simulink model "DisableController"  (Simulink 8.6)
settings: Solver=VariableStepAuto  StartTime=0.0  StopTime=inf  RelTol=1e-3
libraries: simulink_extras x1
settings Model: Creator=Oscar  LastModifiedBy=Oscar
settings DataIOCC: SaveFormat=Dataset  SignalLoggingSaveFormat=Dataset
settings OptimizationCC: ExpressionDepthLimit=128
settings DebuggingCC: UnderspecifiedInitializationDetection=Simplified  MergeDetectMultiDrivingBlocksExec=error  SolverPrmCheckMsg=none  FcnCallInpInsideContextMsg=EnableAllAsError  StateNameClashWarn=none
settings HardwareCC: ProdBitPerPointer=64  ProdLargestAtomicFloat=Float  ProdIntDivRoundTo=Zero  ProdEndianess=LittleEndian  ProdWordSize=64  ProdHWDeviceType=Intel->x86-64 (Windows64)
settings GRTTargetCC: GeneratePreprocessorConditionals=Use local settings  CombineOutputUpdateFcns=on  GRTInterface=off
settings ConfigComp: CovModelRefEnable=off

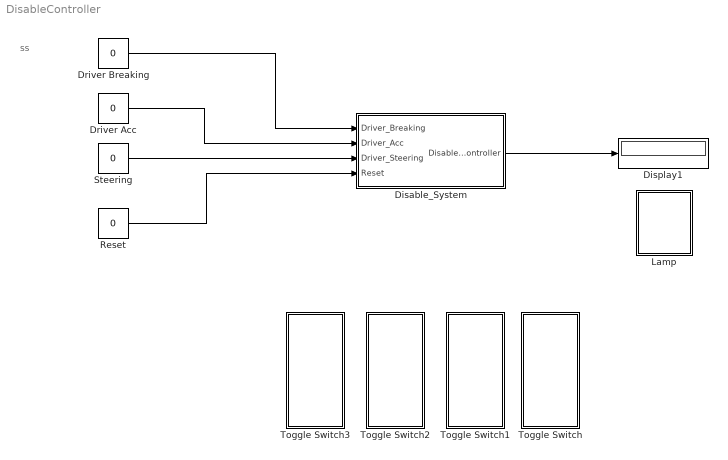
== system DisableController ==
  note: ss
  Disable_System : Subsystem
  Display1 : Display
  Driver Acc : Constant  Value=0
  Driver Breaking : Constant  Value=0
  Lamp : Subsystem  DialogController=hmiCreateDDGDialog  DialogControllerArgs=DataTag0  IsWebBlock=on  mask(MWDashboardBlock){webBlockId=f0d4b18d-8bb7-414d-912f-2697fe4de823, webBlockType=lamp, ShowInLibBrowser=on, ShowInitialText=on, HMISrcModelName=DisableController}
      mask prompts: webBlockType "WebBlock Type"; HMISrcModelName "Source Model"
      mask Help: helpview([docroot '/mapfiles/simulink.map'], 'hmi_lamp')
      mask Display:
      | if strcmp(get_param(bdroot(gcb),'BlockDiagramType'), 'library')
      |     image([(matlabroot) '/toolbox/simulink/hmi/icons/Lamp.png']);
      | end
  Reset : Constant  Value=0
  Steering : Constant  Value=0
  Toggle Switch : Subsystem  DialogController=hmiCreateDDGDialog  DialogControllerArgs=DataTag1  IsWebBlock=on  mask(MWDashboardBlock){webBlockId=8696f94f-6ba7-4cf2-b2c4-95ca151c8475, webBlockType=toggleswitch, ShowInLibBrowser=on, ShowInitialText=on, HMISrcModelName=DisableController}
      mask prompts: webBlockId "WebBlock Id"; webBlockType "WebBlock Type"; HMISrcModelName "Source Model"
      mask Help: helpview([docroot '/mapfiles/simulink.map'], 'hmi_toggle_switch')
      mask Display:
      | if strcmp(get_param(bdroot(gcb),'BlockDiagramType'), 'library')
      |     image([(matlabroot) '/toolbox/simulink/hmi/icons/ToggleSwitch.png']);
      | end
  Toggle Switch1 : Subsystem  DialogController=hmiCreateDDGDialog  DialogControllerArgs=DataTag2  IsWebBlock=on  mask(MWDashboardBlock){webBlockId=361f9ab1-9628-4675-8173-fcd33670bfa1, webBlockType=toggleswitch, ShowInLibBrowser=on, ShowInitialText=on, HMISrcModelName=DisableController}
      mask prompts: webBlockId "WebBlock Id"; webBlockType "WebBlock Type"; HMISrcModelName "Source Model"
      mask Help: helpview([docroot '/mapfiles/simulink.map'], 'hmi_toggle_switch')
      mask Display:
      | if strcmp(get_param(bdroot(gcb),'BlockDiagramType'), 'library')
      |     image([(matlabroot) '/toolbox/simulink/hmi/icons/ToggleSwitch.png']);
      | end
  Toggle Switch2 : Subsystem  DialogController=hmiCreateDDGDialog  DialogControllerArgs=DataTag3  IsWebBlock=on  mask(MWDashboardBlock){webBlockId=eedc1ba2-2433-4e35-ba26-c33148832a6b, webBlockType=toggleswitch, ShowInLibBrowser=on, ShowInitialText=on, HMISrcModelName=DisableController}
      mask prompts: webBlockId "WebBlock Id"; webBlockType "WebBlock Type"; HMISrcModelName "Source Model"
      mask Help: helpview([docroot '/mapfiles/simulink.map'], 'hmi_toggle_switch')
      mask Display:
      | if strcmp(get_param(bdroot(gcb),'BlockDiagramType'), 'library')
      |     image([(matlabroot) '/toolbox/simulink/hmi/icons/ToggleSwitch.png']);
      | end
  Toggle Switch3 : Subsystem  DialogController=hmiCreateDDGDialog  DialogControllerArgs=DataTag4  IsWebBlock=on  mask(MWDashboardBlock){webBlockId=0cae81f2-8a2d-4286-bc79-44c17df7e163, webBlockType=toggleswitch, ShowInLibBrowser=on, ShowInitialText=on, HMISrcModelName=DisableController}
      mask prompts: webBlockId "WebBlock Id"; webBlockType "WebBlock Type"; HMISrcModelName "Source Model"
      mask Help: helpview([docroot '/mapfiles/simulink.map'], 'hmi_toggle_switch')
      mask Display:
      | if strcmp(get_param(bdroot(gcb),'BlockDiagramType'), 'library')
      |     image([(matlabroot) '/toolbox/simulink/hmi/icons/ToggleSwitch.png']);
      | end
  wires:
  Driver Breaking/1 -> Disable_System/1(Driver_Breaking)
  Driver Acc/1 -> Disable_System/2(Driver_Acc)
  Reset/1 -> Disable_System/4(Reset)
  Disable_System/1(Disable_Controller) -> Display1/1
  Steering/1 -> Disable_System/3(Driver_Steering)

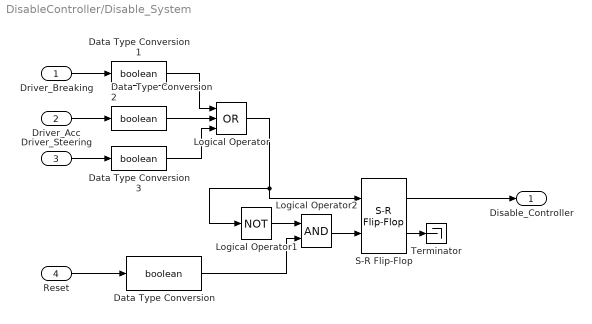
== system DisableController/Disable_System ==
  Driver_Breaking : Inport
  Driver_Acc : Inport  Port=2
  Driver_Steering : Inport  Port=3
  Reset : Inport  Port=4
  Data Type Conversion{,1..3} (4 alike) : DataTypeConversion  OutDataTypeStr=boolean
  Logical Operator : Logic  Operator=OR  Inputs=3  AllPortsSameDT=off  OutDataTypeStr=boolean
  Logical Operator1 : Logic  Operator=NOT  AllPortsSameDT=off  OutDataTypeStr=boolean
  Logical Operator2 : Logic  AllPortsSameDT=off  OutDataTypeStr=boolean
  S-R Flip-Flop : simulink_extras/Flip Flops/S-R Flip-Flop  initial_condition=0
  Terminator : Terminator
  Disable_Controller : Outport
  wires:
  Logical Operator1/1 -> Logical Operator2/1
  Driver_Acc/1 -> Data Type Conversion2/1
  S-R Flip-Flop/1 -> Disable_Controller/1
  Logical Operator/1 -> S-R Flip-Flop/1, Logical Operator1/1
  S-R Flip-Flop/2 -> Terminator/1
  Driver_Breaking/1 -> Data Type Conversion1/1
  Reset/1 -> Data Type Conversion/1
  Data Type Conversion/1 -> Logical Operator2/2
  Logical Operator2/1 -> S-R Flip-Flop/2
  Driver_Steering/1 -> Data Type Conversion3/1
  Data Type Conversion1/1 -> Logical Operator/1
  Data Type Conversion2/1 -> Logical Operator/2
  Data Type Conversion3/1 -> Logical Operator/3

== system DisableController/Lamp ==

== system DisableController/Toggle Switch ==

== system DisableController/Toggle Switch1 ==

== system DisableController/Toggle Switch2 ==

== system DisableController/Toggle Switch3 ==
